simulink model "flightController"  (R2021a)
settings: Solver=ode3  StartTime=0  StopTime=TFinal  FixedStep=Ts  RelTol=1e-3  EnableMultiTasking=on
undefined symbols (not defined in the file): Controller, DiscIntNeverNeededParam, g, K, KLQI, KLQR, linsys, NBar, Ts, Vehicle
settings Model: ExtModeTrigDuration=80  Creator=The MathWorks, Inc.  LastModifiedBy=House
settings SolverCC: AlgebraicLoopSolver=TrustRegion  MinimalZcImpactIntegration=on
settings DataIOCC: LimitDataPoints=on  ReturnWorkspaceOutputs=off
settings OptimizationCC: BlockReduction=off  EnhancedBackFolding=on  PassReuseOutputArgsAs=Individual arguments  ZeroExternalMemoryAtStartup=off  ZeroInternalMemoryAtStartup=off  MaxStackSize=64  OptimizeBlockOrder=speed  DifferentSizesBufferReuse=on  OptimizationCustomize=off  EfficientTunableParamExpr=on
settings DebuggingCC: AlgebraicLoopMsg=none  ParameterPrecisionLossMsg=none  ParameterTunabilityLossMsg=error  UnconnectedInputMsg=none  UnconnectedOutputMsg=none  UnconnectedLineMsg=none  BusObjectLabelMismatch=error  SFUnexpectedBacktrackingDiag=warning  SFNoUnconditionalDefaultTransitionDiag=warning  SFExecutionAtInitializationDiag=none  SFMachineParentedDataDiag=warning  ArithmeticOperatorsInVariantConditions=warning
settings HardwareCC: ProdBitPerPointer=32  ProdBitPerSizeT=32  ProdBitPerPtrDiffT=32  ProdLargestAtomicInteger=Long  ProdWordSize=32  ProdHWDeviceType=ARM Compatible->ARM 9
settings ModelReferenceCC: ModelReferenceNumInstancesAllowed=Single  PropagateSignalLabelsOutOfModel=off
settings SFSimCC: SimUseLocalCustomCode=off  MATLABDynamicMemAlloc=off  CustomCodeUndefinedFunction=UseInterfaceOnly
settings RTWCC: SystemTargetFile=ert.tlc  HardwareBoard=PARROT Mambo  TemplateMakefile=ert_default_tmf  GenerateReport=on  RTWUseLocalCustomCode=off  Toolchain=Sourcery G++ Lite GNU Toolchain for Drones  LaunchReport=on
settings CodeAppCC: ForceParamTrailComments=on  IgnoreCustomStorageClasses=off  MaxIdLength=63  OperatorAnnotations=on  SimulinkDataObjDesc=on  SFDataObjDesc=on  InsertBlockDesc=on
settings ERTTargetCC: MatFileLogging=on
settings ConfigComp: CovMetricSettings=dw  CovSaveCumulativeToWorkspaceVar=on  CovSaveSingleToWorkspaceVar=on  CovExternalEMLEnable=off  CovSFcnEnable=off

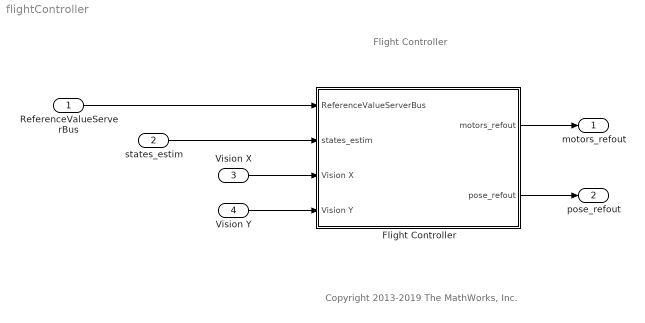
== system flightController ==
  note: Flight Controller
  note: Copyright 2013-2019 The MathWorks, Inc.
  ReferenceValueServerBus : Inport  OutDataTypeStr=Bus: CommandBus  BusOutputAsStruct=on
  states_estim : Inport  Port=2  OutDataTypeStr=Bus: statesEstim_t  BusOutputAsStruct=on
  Vision X : Inport  Port=3
  Vision Y : Inport  Port=4
  Flight Controller : Subsystem
  motors_refout : Outport  VectorParamsAs1DForOutWhenUnconnected=off
  pose_refout : Outport  Port=2  VectorParamsAs1DForOutWhenUnconnected=off
  wires:
  ReferenceValueServerBus/1 -> Flight Controller/1(ReferenceValueServerBus)
  states_estim/1 -> Flight Controller/2(states_estim)
  Flight Controller/2(pose_refout) -> pose_refout/1
  Flight Controller/1(motors_refout) -> motors_refout/1
  Vision X/1 -> Flight Controller/3(Vision X)
  Vision Y/1 -> Flight Controller/4(Vision Y)

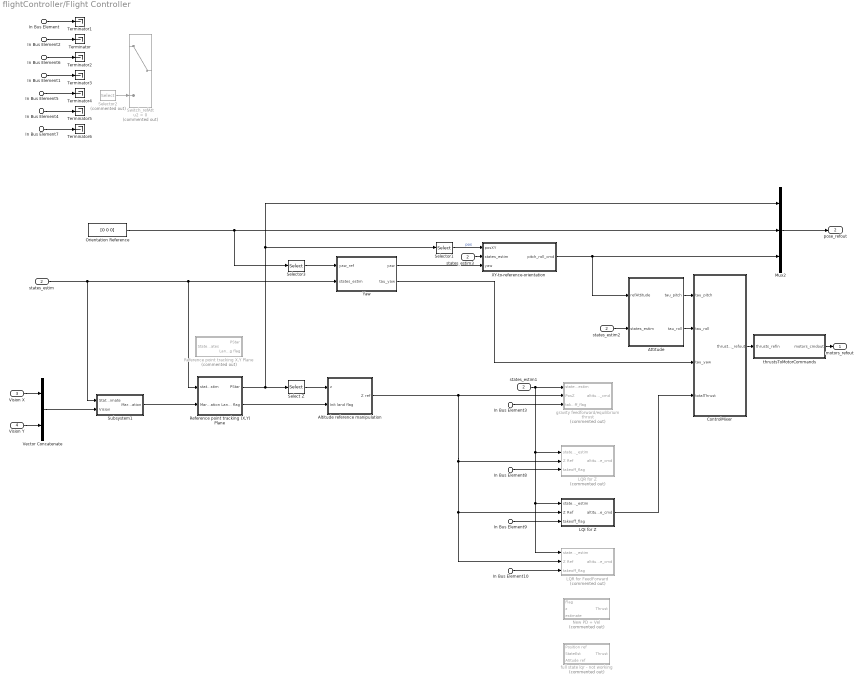
== system flightController/Flight Controller ==
  In Bus Element1 : Inport  PortName=ReferenceValueServerBus  Element=controlModePosVSOrient
  In Bus Element : Inport  PortName=ReferenceValueServerBus  Element=pos_ref
  In Bus Element4 : Inport  PortName=ReferenceValueServerBus  Element=pos_ref
  In Bus Element5 : Inport  PortName=ReferenceValueServerBus  Element=pos_ref
  In Bus Element2 : Inport  PortName=ReferenceValueServerBus  Element=orient_ref
  In Bus Element6 : Inport  PortName=ReferenceValueServerBus  Element=orient_ref
  In Bus Element7 : Inport  PortName=ReferenceValueServerBus  Element=orient_ref
  In Bus Element{3,8..10} (4 alike) : Inport  PortName=ReferenceValueServerBus  Element=takeoff_flag
  states_estim : Inport  Port=2
  Vision X : Inport  Port=3
  Vision Y : Inport  Port=4
  Altitude reference manipulation : Subsystem
  Attitude : Subsystem
  ControlMixer : Subsystem
  LQI for Z : Subsystem
  LQR for FeedForward : Subsystem  Commented=on
  LQR for Z : Subsystem  Commented=on
  Mux2 : Mux  Inputs=3
  New PD + Vel : Subsystem  Commented=on
  Orientation Reference : Constant  Value=[0 0 0]  OutDataTypeStr=single
  Reference point tracking (X,Y) Plane : Subsystem
  Reference point tracking X,Y Plane : Subsystem  Commented=on
  Select Z : Selector  InputPortWidth=3  IndexOptions=Index vector (dialog)  Indices=3  OutputSizes=1
  Selector1 : Selector  InputPortWidth=3  IndexOptions=Index vector (dialog)  Indices=[1 2]  OutputSizes=1
  Selector2 : Selector  Commented=on  InputPortWidth=3  IndexOptions=Index vector (dialog)  Indices=[2 3]  OutputSizes=1
  Selector3 : Selector  InputPortWidth=3  IndexOptions=Index vector (dialog)  Indices=1  OutputSizes=1
  Subsystem1 : Subsystem
  Switch_refAtt : Switch  Commented=on  Criteria=u2 > Threshold
  Terminator{,1..6} (7 alike) : Terminator
  Vector Concatenate : Concatenate
  XY-to-reference-orientation : Subsystem
  Yaw : Subsystem
  full state lqr - not working : Subsystem  Commented=on
  gravity feedforward/equilibrium thrust : Subsystem  Commented=on
  states_estim1 : InportShadow  Port=2
  states_estim2 : InportShadow  Port=2
  states_estim3 : InportShadow  Port=2
  thrustsToMotorCommands : Subsystem
  motors_refout : Outport  VectorParamsAs1DForOutWhenUnconnected=off
  pose_refout : Outport  Port=2  VectorParamsAs1DForOutWhenUnconnected=off
  wires:
  thrustsToMotorCommands/1(motors_cmdout) -> motors_refout/1
  Selector3/1 -> Yaw/1(yaw_ref)
  Selector1/1 -> XY-to-reference-orientation/1(posXY)  "pos"
  ControlMixer/1(thrusts_refout) -> thrustsToMotorCommands/1(thrusts_refin)
  In Bus Element3/1 -> gravity feedforward/equilibrium thrust/3(takeoff_flag)
  states_estim/1 -> Subsystem1/1(State Estimate), Reference point tracking (X,Y) Plane/1(states_estim), Yaw/2(states_estim)
  Yaw/1(yaw) -> XY-to-reference-orientation/3(yaw)
  Mux2/1 -> pose_refout/1
  Attitude/1(tau_pitch) -> ControlMixer/1(tau_pitch)
  Attitude/2(tau_roll) -> ControlMixer/2(tau_roll)
  Yaw/2(tau_yaw) -> ControlMixer/3(tau_yaw)
  states_estim1/1 -> LQR for FeedForward/1(states_estim), LQI for Z/1(states_estim), LQR for Z/1(states_estim), gravity feedforward/equilibrium thrust/1(states_estim)
  states_estim2/1 -> Attitude/2(states_estim)
  states_estim3/1 -> XY-to-reference-orientation/2(states_estim)
  Selector2/1 -> Switch_refAtt/3
  In Bus Element2/1 -> Terminator/1
  In Bus Element/1 -> Terminator1/1
  In Bus Element6/1 -> Terminator2/1
  In Bus Element1/1 -> Terminator3/1
  In Bus Element5/1 -> Terminator4/1
  XY-to-reference-orientation/1(pitch_roll_cmd) -> Attitude/1(refAttitude), Mux2/3
  In Bus Element4/1 -> Terminator5/1
  Orientation Reference/1 -> Selector3/1, Mux2/2
  In Bus Element7/1 -> Terminator6/1
  Altitude reference manipulation/1(Z ref) -> LQR for FeedForward/2(Z Ref), LQI for Z/2(Z Ref), LQR for Z/2(Z Ref), gravity feedforward/equilibrium thrust/2(PosZ)
  In Bus Element8/1 -> LQR for Z/3(takeoff_flag)
  In Bus Element9/1 -> LQI for Z/3(takeoff_flag)
  In Bus Element10/1 -> LQR for FeedForward/3(takeoff_flag)
  Select Z/1 -> Altitude reference manipulation/1(z)
  Reference point tracking (X,Y) Plane/1(PStar) -> Selector1/1, Mux2/1, Select Z/1
  Reference point tracking (X,Y) Plane/2(Landing flag) -> Altitude reference manipulation/2(Init land flag)
  Vision X/1 -> Vector Concatenate/1
  Vision Y/1 -> Vector Concatenate/2
  Vector Concatenate/1 -> Subsystem1/2(Vision)
  Subsystem1/1(Marker Location) -> Reference point tracking (X,Y) Plane/2(Marker Location)
  LQI for Z/1(altitude_cmd) -> ControlMixer/4(totalThrust)

== system flightController/Flight Controller/Altitude reference manipulation ==
  z : Inport
  Init land flag : Inport  Port=2
  Constant3 : Constant  Value=Ts  OutDataTypeStr=single
  Delay : Delay  DelayLength=600
  Landing spline : Scope  NumInputPorts=2
  Landing spline Dependent on time - works : MATLAB Function  TreatAsAtomicUnit=on
  Landing spline Dependent on time - works My version : MATLAB Function  Commented=on  TreatAsAtomicUnit=on
  Memory : Memory
  Switch : Switch  Criteria=u2 > Threshold
  Z ref : Outport
  wires:
  Constant3/1 -> Landing spline Dependent on time - works/2(time)
  Delay/1 -> Landing spline Dependent on time - works/3(flag)
  Landing spline Dependent on time - works/1(ZdOut) -> Landing spline/2, Z ref/1
  Init land flag/1 -> Switch/2, Delay/1
  z/1 -> Switch/3
  Switch/1 -> Memory/1, Landing spline/1, Landing spline Dependent on time - works/1(z)
  Memory/1 -> Switch/1

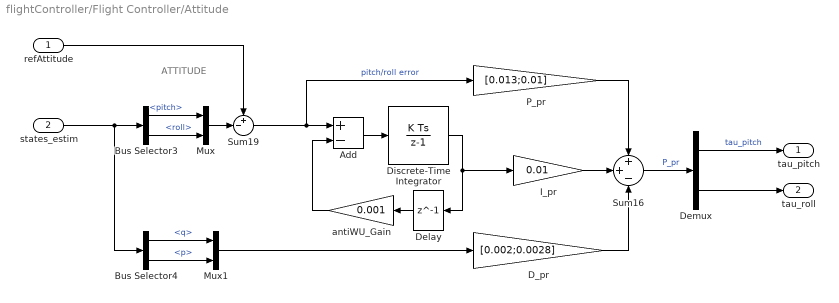
== system flightController/Flight Controller/Attitude ==
  note: ATTITUDE
  refAttitude : Inport
  states_estim : Inport  Port=2
  Add : Sum  Inputs=+-
  Bus Selector3 : BusSelector  OutputSignals=pitch,roll
  Bus Selector4 : BusSelector  OutputSignals=q,p
  D_pr : Gain  Gain=[0.002;0.0028]
  Delay : Delay  DelayLength=1  InitialCondition=0
  Demux : Demux  Outputs=2
  Discrete-Time Integrator : DiscreteIntegrator  SampleTime=Ts  LimitOutput=on  UpperSaturationLimit=2  LowerSaturationLimit=-2  ICPrevOutput=DiscIntNeverNeededParam  ICPrevScaledInput=DiscIntNeverNeededParam
  I_pr : Gain  Gain=0.01
  Mux : Mux  Inputs=2
  Mux1 : Mux  Inputs=2
  P_pr : Gain  Gain=[0.013;0.01]
  Sum16 : Sum  Inputs=++-  AccumDataTypeStr=single  OutDataTypeStr=single  SaturateOnIntegerOverflow=on
  Sum19 : Sum  Inputs=+-|
  antiWU_Gain : Gain  Gain=0.001
  tau_pitch : Outport  VectorParamsAs1DForOutWhenUnconnected=off
  tau_roll : Outport  Port=2  VectorParamsAs1DForOutWhenUnconnected=off
  wires:
  Sum16/1 -> Demux/1  "P_pr"
  antiWU_Gain/1 -> Add/2
  Add/1 -> Discrete-Time Integrator/1
  Bus Selector3/1 -> Mux/1  "<pitch>"
  Bus Selector4/1 -> Mux1/1  "<q>"
  P_pr/1 -> Sum16/1
  I_pr/1 -> Sum16/2
  Sum19/1 -> Add/1, P_pr/1  "pitch/roll error"
  Discrete-Time Integrator/1 -> Delay/1, I_pr/1
  Delay/1 -> antiWU_Gain/1
  Demux/1 -> tau_pitch/1  "tau_pitch"
  Demux/2 -> tau_roll/1
  D_pr/1 -> Sum16/3
  states_estim/1 -> Bus Selector3/1, Bus Selector4/1
  refAttitude/1 -> Sum19/1
  Mux/1 -> Sum19/2
  Bus Selector3/2 -> Mux/2  "<roll>"
  Mux1/1 -> D_pr/1
  Bus Selector4/2 -> Mux1/2  "<p>"

== system flightController/Flight Controller/ControlMixer ==
  tau_pitch : Inport
  tau_roll : Inport  Port=2
  tau_yaw : Inport  Port=3
  totalThrust : Inport  Port=4
  Mux2 : Mux
  Product : Product  Multiplication=Matrix(*)  RndMeth=Zero
  TorqueTotalThrustToThrustPerMotor : Constant  Value=Controller.Q2Ts  OutDataTypeStr=single
  thrusts_refout : Outport  VectorParamsAs1DForOutWhenUnconnected=off
  wires:
  Product/1 -> thrusts_refout/1
  tau_roll/1 -> Mux2/4
  tau_pitch/1 -> Mux2/3
  tau_yaw/1 -> Mux2/2
  totalThrust/1 -> Mux2/1
  TorqueTotalThrustToThrustPerMotor/1 -> Product/1
  Mux2/1 -> Product/2

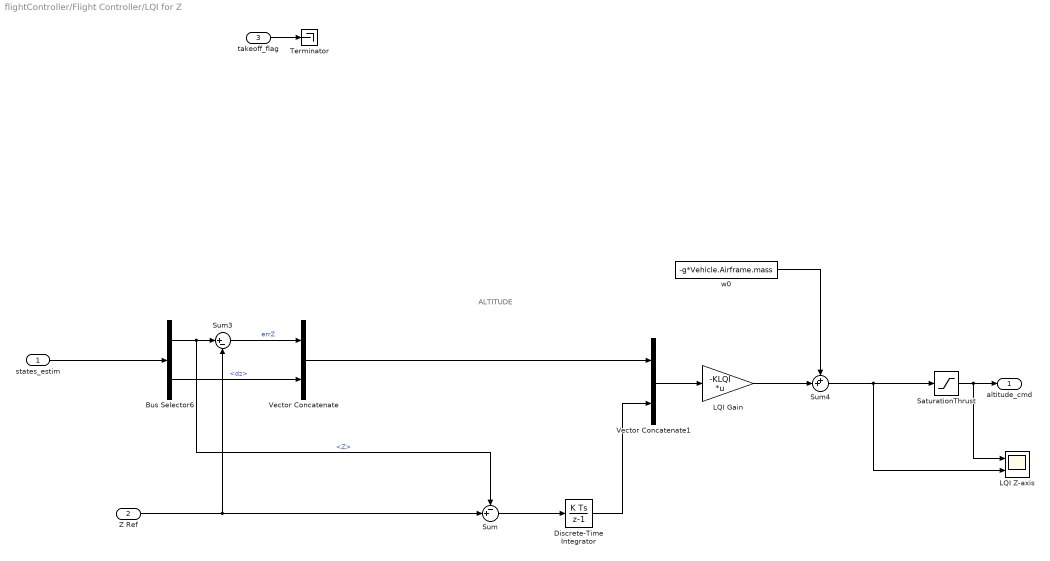
== system flightController/Flight Controller/LQI for Z ==
  note: ALTITUDE
  states_estim : Inport
  Z Ref : Inport  Port=2
  takeoff_flag : Inport  Port=3
  Bus Selector6 : BusSelector  OutputSignals=Z,dz
  Discrete-Time Integrator : DiscreteIntegrator  SampleTime=-1  ICPrevOutput=DiscIntNeverNeededParam  ICPrevScaledInput=DiscIntNeverNeededParam
  LQI Gain : Gain  Gain=-KLQI  Multiplication=Matrix(K*u) (u vector)
  LQI Z-axis : Scope  NumInputPorts=2
  SaturationThrust : Saturate  UpperLimit=4*Controller.totalThrustMaxRelative*Controller.motorsThrustPerMotorMax  LowerLimit=-4*Controller.totalThrustMaxRelative*Controller.motorsThrustPerMotorMax  OutDataTypeStr=single
  Sum : Sum  Inputs=-+|
  Sum3 : Sum  Inputs=|+-  AccumDataTypeStr=single  OutDataTypeStr=single  SaturateOnIntegerOverflow=on
  Sum4 : Sum  Inputs=++|  AccumDataTypeStr=single  OutDataTypeStr=single  SaturateOnIntegerOverflow=on
  Terminator : Terminator
  Vector Concatenate : Concatenate
  Vector Concatenate1 : Concatenate
  w0 : Constant  Value=-g*Vehicle.Airframe.mass  OutDataTypeStr=single  SampleTime=Ts
  altitude_cmd : Outport  VectorParamsAs1DForOutWhenUnconnected=off
  wires:
  states_estim/1 -> Bus Selector6/1
  Sum4/1 -> LQI Z-axis/2, SaturationThrust/1
  w0/1 -> Sum4/1
  SaturationThrust/1 -> LQI Z-axis/1, altitude_cmd/1
  Bus Selector6/2 -> Vector Concatenate/2  "<dz>"
  takeoff_flag/1 -> Terminator/1
  Sum3/1 -> Vector Concatenate/1  "errZ"
  LQI Gain/1 -> Sum4/2
  Vector Concatenate1/1 -> LQI Gain/1
  Vector Concatenate/1 -> Vector Concatenate1/1
  Discrete-Time Integrator/1 -> Vector Concatenate1/2
  Z Ref/1 -> Sum3/2, Sum/2
  Sum/1 -> Discrete-Time Integrator/1
  Bus Selector6/1 -> Sum/1, Sum3/1  "<Z>"

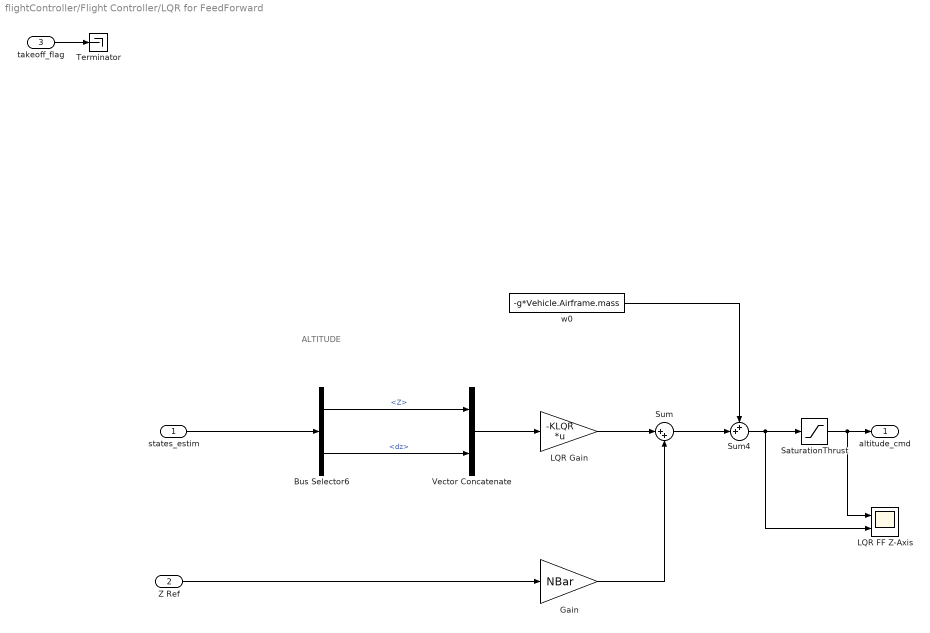
== system flightController/Flight Controller/LQR for FeedForward ==
  note: ALTITUDE
  states_estim : Inport
  Z Ref : Inport  Port=2
  takeoff_flag : Inport  Port=3
  Bus Selector6 : BusSelector  OutputSignals=Z,dz
  Gain : Gain  Gain=NBar
  LQR FF Z-Axis : Scope  NumInputPorts=2
  LQR Gain : Gain  Gain=-KLQR  Multiplication=Matrix(K*u) (u vector)
  SaturationThrust : Saturate  UpperLimit=4*Controller.totalThrustMaxRelative*Controller.motorsThrustPerMotorMax  LowerLimit=-4*Controller.totalThrustMaxRelative*Controller.motorsThrustPerMotorMax  OutDataTypeStr=single
  Sum : Sum  Inputs=|++
  Sum4 : Sum  Inputs=++|  AccumDataTypeStr=single  OutDataTypeStr=single  SaturateOnIntegerOverflow=on
  Terminator : Terminator
  Vector Concatenate : Concatenate
  w0 : Constant  Value=-g*Vehicle.Airframe.mass  OutDataTypeStr=single  SampleTime=Ts
  altitude_cmd : Outport  VectorParamsAs1DForOutWhenUnconnected=off
  wires:
  states_estim/1 -> Bus Selector6/1
  Sum4/1 -> LQR FF Z-Axis/2, SaturationThrust/1
  SaturationThrust/1 -> LQR FF Z-Axis/1, altitude_cmd/1
  Bus Selector6/2 -> Vector Concatenate/2  "<dz>"
  takeoff_flag/1 -> Terminator/1
  Vector Concatenate/1 -> LQR Gain/1
  Z Ref/1 -> Gain/1
  Bus Selector6/1 -> Vector Concatenate/1  "<Z>"
  w0/1 -> Sum4/1
  LQR Gain/1 -> Sum/1
  Sum/1 -> Sum4/2
  Gain/1 -> Sum/2

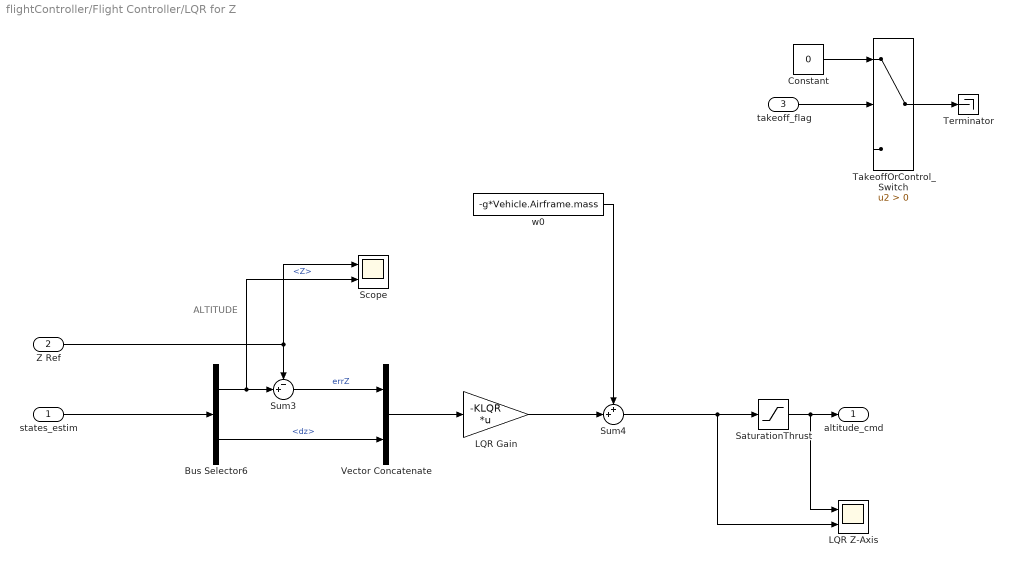
== system flightController/Flight Controller/LQR for Z ==
  note: ALTITUDE
  states_estim : Inport
  Z Ref : Inport  Port=2
  takeoff_flag : Inport  Port=3
  Bus Selector6 : BusSelector  OutputSignals=Z,dz
  Constant : Constant  Value=0  OutDataTypeStr=single
  LQR Gain : Gain  Gain=-KLQR  Multiplication=Matrix(K*u) (u vector)
  LQR Z-Axis : Scope  NumInputPorts=2
  SaturationThrust : Saturate  UpperLimit=4*Controller.totalThrustMaxRelative*Controller.motorsThrustPerMotorMax  LowerLimit=-4*Controller.totalThrustMaxRelative*Controller.motorsThrustPerMotorMax  OutDataTypeStr=single
  Scope : Scope  NumInputPorts=2
  Sum3 : Sum  Inputs=-+|  AccumDataTypeStr=single  OutDataTypeStr=single  SaturateOnIntegerOverflow=on
  Sum4 : Sum  Inputs=++|  AccumDataTypeStr=single  OutDataTypeStr=single  SaturateOnIntegerOverflow=on
  TakeoffOrControl_Switch : Switch  Criteria=u2 > Threshold
  Terminator : Terminator
  Vector Concatenate : Concatenate
  w0 : Constant  Value=-g*Vehicle.Airframe.mass  OutDataTypeStr=single  SampleTime=Ts
  altitude_cmd : Outport  VectorParamsAs1DForOutWhenUnconnected=off
  wires:
  states_estim/1 -> Bus Selector6/1
  Sum4/1 -> LQR Z-Axis/2, SaturationThrust/1
  w0/1 -> Sum4/1
  SaturationThrust/1 -> altitude_cmd/1, LQR Z-Axis/1
  Bus Selector6/2 -> Vector Concatenate/2  "<dz>"
  Bus Selector6/1 -> Scope/2, Sum3/2  "<Z>"
  Z Ref/1 -> Sum3/1, Scope/1
  Sum3/1 -> Vector Concatenate/1  "errZ"
  Vector Concatenate/1 -> LQR Gain/1
  LQR Gain/1 -> Sum4/2
  Constant/1 -> TakeoffOrControl_Switch/1
  takeoff_flag/1 -> TakeoffOrControl_Switch/2
  TakeoffOrControl_Switch/1 -> Terminator/1

== system flightController/Flight Controller/New PD + Vel ==
  Flag : Inport
  z : Inport  Port=2
  estimate : Inport  Port=3
  Altitude reference manipulation With Velocity calculation : Subsystem
  gravity feedforward/equilibrium thrust : Subsystem
  Thrust : Outport
  wires:
  Flag/1 -> Altitude reference manipulation With Velocity calculation/1(Init land flag)
  z/1 -> Altitude reference manipulation With Velocity calculation/2(z)
  estimate/1 -> gravity feedforward/equilibrium thrust/1(states_estim), Altitude reference manipulation With Velocity calculation/3(State estimate)
  Altitude reference manipulation With Velocity calculation/1(Z ref) -> gravity feedforward/equilibrium thrust/2(PosZ)
  gravity feedforward/equilibrium thrust/1(altitude_cmd) -> Thrust/1

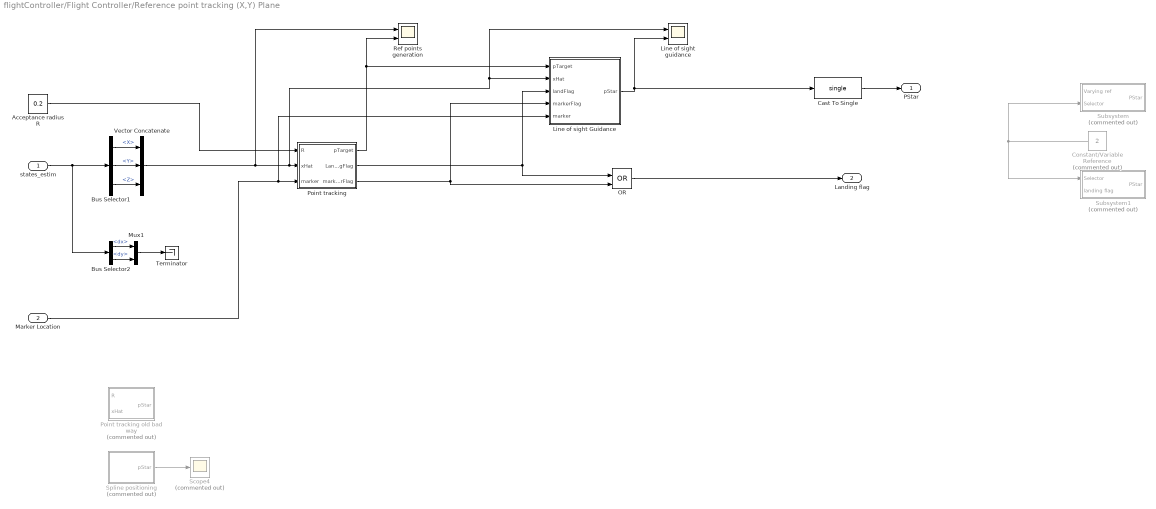
== system flightController/Flight Controller/Reference point tracking (X,Y) Plane ==
  states_estim : Inport
  Marker Location : Inport  Port=2
  Acceptance radius R : Constant  Value=0.2  OutDataTypeStr=single
  Bus Selector1 : BusSelector  OutputSignals=X,Y,Z
  Bus Selector2 : BusSelector  OutputSignals=dx,dy
  Cast To Single : DataTypeConversion  OutDataTypeStr=single
  Constant/Variable Reference : Constant  Commented=on  Value=2  OutDataTypeStr=single
  Line of sight Guidance : MATLAB Function  TreatAsAtomicUnit=on
  Line of sight guidance : Scope  NumInputPorts=2
  Mux1 : Mux  Inputs=2
  OR : Logic  Operator=OR  IconShape=distinctive  AllPortsSameDT=off  OutDataTypeStr=boolean
  Point tracking : MATLAB Function  TreatAsAtomicUnit=on
  Point tracking old bad way : MATLAB Function  Commented=on  TreatAsAtomicUnit=on
  Ref points generation : Scope  NumInputPorts=2
  Scope4 : Scope  Commented=on
  Spline positioning : MATLAB Function  Commented=on  TreatAsAtomicUnit=on
  Subsystem : Subsystem  Commented=on
  Subsystem1 : Subsystem  Commented=on
  Terminator : Terminator
  Vector Concatenate : Concatenate  NumInputs=3
  PStar : Outport
  Landing flag : Outport  Port=2
  wires:
  Bus Selector2/1 -> Mux1/1  "<dx>"
  states_estim/1 -> Bus Selector2/1, Bus Selector1/1
  Bus Selector1/2 -> Vector Concatenate/2  "<Y>"
  Bus Selector1/3 -> Vector Concatenate/3  "<Z>"
  Bus Selector1/1 -> Vector Concatenate/1  "<X>"
  Bus Selector2/2 -> Mux1/2  "<dy>"
  Mux1/1 -> Terminator/1
  Spline positioning/1(pStar) -> Scope4/1
  Line of sight Guidance/1(pStar) -> Cast To Single/1, Line of sight guidance/2
  Constant/Variable Reference/1 -> Subsystem1/1(Selector), Subsystem/2(Selector)
  Cast To Single/1 -> PStar/1
  Point tracking/1(pTarget) -> Ref points generation/2, Line of sight Guidance/1(pTarget)
  Vector Concatenate/1 -> Ref points generation/1, Line of sight guidance/1, Line of sight Guidance/2(xHat), Point tracking/2(xHat)
  Acceptance radius R/1 -> Point tracking/1(R)
  Point tracking/2(LandingFlag) -> OR/1, Line of sight Guidance/3(landFlag)
  Marker Location/1 -> Line of sight Guidance/5(marker), Point tracking/3(marker)
  Point tracking/3(markerFlag) -> OR/2, Line of sight Guidance/4(markerFlag)
  OR/1 -> Landing flag/1

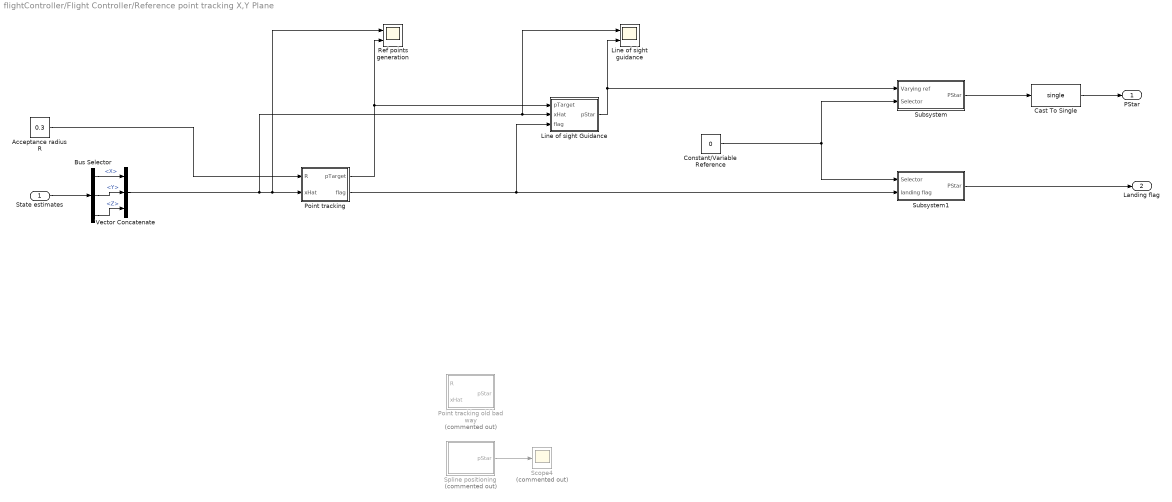
== system flightController/Flight Controller/Reference point tracking X,Y Plane ==
  State estimates : Inport
  Acceptance radius R : Constant  Value=0.3
  Bus Selector : BusSelector  OutputSignals=X,Y,Z
  Cast To Single : DataTypeConversion  OutDataTypeStr=single
  Constant/Variable Reference : Constant  Value=0
  Line of sight Guidance : MATLAB Function  TreatAsAtomicUnit=on
  Line of sight guidance : Scope  NumInputPorts=2
  Point tracking : MATLAB Function  TreatAsAtomicUnit=on
  Point tracking old bad way : MATLAB Function  Commented=on  TreatAsAtomicUnit=on
  Ref points generation : Scope  NumInputPorts=2
  Scope4 : Scope  Commented=on
  Spline positioning : MATLAB Function  Commented=on  TreatAsAtomicUnit=on
  Subsystem : Subsystem
  Subsystem1 : Subsystem
  Vector Concatenate : Concatenate  NumInputs=3
  PStar : Outport
  Landing flag : Outport  Port=2
  wires:
  Bus Selector/3 -> Vector Concatenate/3  "<Z>"
  Bus Selector/1 -> Vector Concatenate/1  "<X>"
  Point tracking/1(pTarget) -> Line of sight Guidance/1(pTarget), Ref points generation/2
  Acceptance radius R/1 -> Point tracking/1(R)
  Bus Selector/2 -> Vector Concatenate/2  "<Y>"
  Vector Concatenate/1 -> Line of sight guidance/1, Line of sight Guidance/2(xHat), Ref points generation/1, Point tracking/2(xHat)
  Line of sight Guidance/1(pStar) -> Subsystem/1(Varying ref), Line of sight guidance/2
  Point tracking/2(flag) -> Subsystem1/2(landing flag), Line of sight Guidance/3(flag)
  State estimates/1 -> Bus Selector/1
  Spline positioning/1(pStar) -> Scope4/1
  Constant/Variable Reference/1 -> Subsystem1/1(Selector), Subsystem/2(Selector)
  Subsystem/1(PStar) -> Cast To Single/1
  Subsystem1/1(PStar) -> Landing flag/1
  Cast To Single/1 -> PStar/1

== system flightController/Flight Controller/Subsystem1 ==
  State Estimate : Inport
  Vision : Inport  Port=2
  Bus Selector6 : BusSelector  OutputSignals=Z
  Constant : Constant  Value=0.004  OutDataTypeStr=single
  Display : Display
  Display1 : Display
  Display2 : Display
  Divide : Product  Inputs=**
  Divide1 : Product  Inputs=**
  Gain : Gain  OutDataTypeStr=Inherit: Same as input
  Marker Location : Outport
  wires:
  State Estimate/1 -> Bus Selector6/1
  Bus Selector6/1 -> Divide/2, Display2/1  "<Z>"
  Constant/1 -> Divide/1
  Divide/1 -> Divide1/2
  Vision/1 -> Display/1, Divide1/1
  Divide1/1 -> Gain/1
  Gain/1 -> Display1/1, Marker Location/1

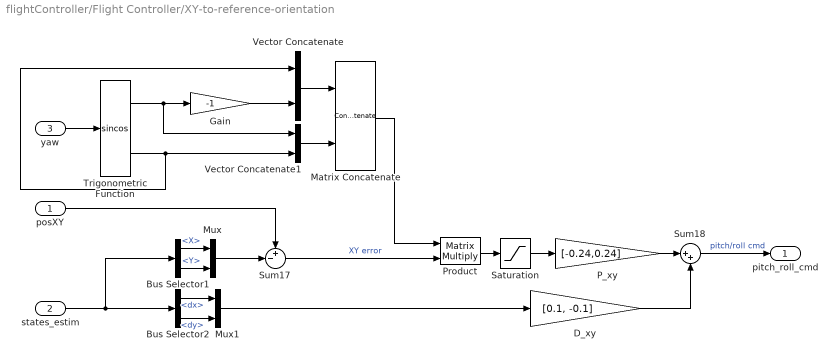
== system flightController/Flight Controller/XY-to-reference-orientation ==
  posXY : Inport
  states_estim : Inport  Port=2
  yaw : Inport  Port=3
  Bus Selector1 : BusSelector  OutputSignals=X,Y
  Bus Selector2 : BusSelector  OutputSignals=dx,dy
  D_xy : Gain  Gain=[0.1, -0.1]  ParamDataTypeStr=single  OutDataTypeStr=single  SaturateOnIntegerOverflow=on
  Gain : Gain  Gain=-1
  Matrix Concatenate : Concatenate  Mode=Multidimensional array  ConcatenateDimension=2
  Mux : Mux  Inputs=2
  Mux1 : Mux  Inputs=2
  P_xy : Gain  Gain=[-0.24,0.24]  ParamDataTypeStr=single  OutDataTypeStr=single  SaturateOnIntegerOverflow=on
  Product : Product  Multiplication=Matrix(*)  OutDataTypeStr=single  RndMeth=Zero
  Saturation : Saturate  UpperLimit=3  LowerLimit=-3  OutDataTypeStr=single
  Sum17 : Sum  Inputs=+-|  AccumDataTypeStr=single
  Sum18 : Sum  Inputs=|++  AccumDataTypeStr=single  OutDataTypeStr=single  SaturateOnIntegerOverflow=on
  Trigonometric Function : Trigonometry  Operator=sincos
  Vector Concatenate : Concatenate
  Vector Concatenate1 : Concatenate
  pitch_roll_cmd : Outport  VectorParamsAs1DForOutWhenUnconnected=off
  wires:
  yaw/1 -> Trigonometric Function/1
  Saturation/1 -> P_xy/1
  P_xy/1 -> Sum18/1
  Sum17/1 -> Product/2  "XY error"
  posXY/1 -> Sum17/1
  Bus Selector2/1 -> Mux1/1  "<dx>"
  states_estim/1 -> Bus Selector1/1, Bus Selector2/1
  Sum18/1 -> pitch_roll_cmd/1  "pitch/roll cmd"
  D_xy/1 -> Sum18/2
  Bus Selector1/1 -> Mux/1  "<X>"
  Product/1 -> Saturation/1
  Trigonometric Function/1 -> Gain/1, Vector Concatenate1/1
  Trigonometric Function/2 -> Vector Concatenate1/2, Vector Concatenate/1
  Gain/1 -> Vector Concatenate/2
  Vector Concatenate/1 -> Matrix Concatenate/1
  Vector Concatenate1/1 -> Matrix Concatenate/2
  Matrix Concatenate/1 -> Product/1
  Bus Selector1/2 -> Mux/2  "<Y>"
  Mux/1 -> Sum17/2
  Mux1/1 -> D_xy/1
  Bus Selector2/2 -> Mux1/2  "<dy>"

== system flightController/Flight Controller/Yaw ==
  yaw_ref : Inport
  states_estim : Inport  Port=2
  Bus Selector5 : BusSelector  OutputSignals=yaw,r
  D_yaw : Gain  Gain=0.3*0.004
  P_yaw : Gain  Gain=0.004  ParamDataTypeStr=single  OutDataTypeStr=single
  Sum1 : Sum  Inputs=+-|  AccumDataTypeStr=single  OutDataTypeStr=single  SaturateOnIntegerOverflow=on
  Sum2 : Sum  Inputs=|+-
  yaw : Outport  VectorParamsAs1DForOutWhenUnconnected=off
  tau_yaw : Outport  Port=2  VectorParamsAs1DForOutWhenUnconnected=off
  wires:
  D_yaw/1 -> Sum2/2
  P_yaw/1 -> Sum2/1
  Bus Selector5/2 -> D_yaw/1  "<r>"
  Sum1/1 -> P_yaw/1
  states_estim/1 -> Bus Selector5/1
  Sum2/1 -> tau_yaw/1
  Bus Selector5/1 -> yaw/1, Sum1/2  "<yaw>"
  yaw_ref/1 -> Sum1/1

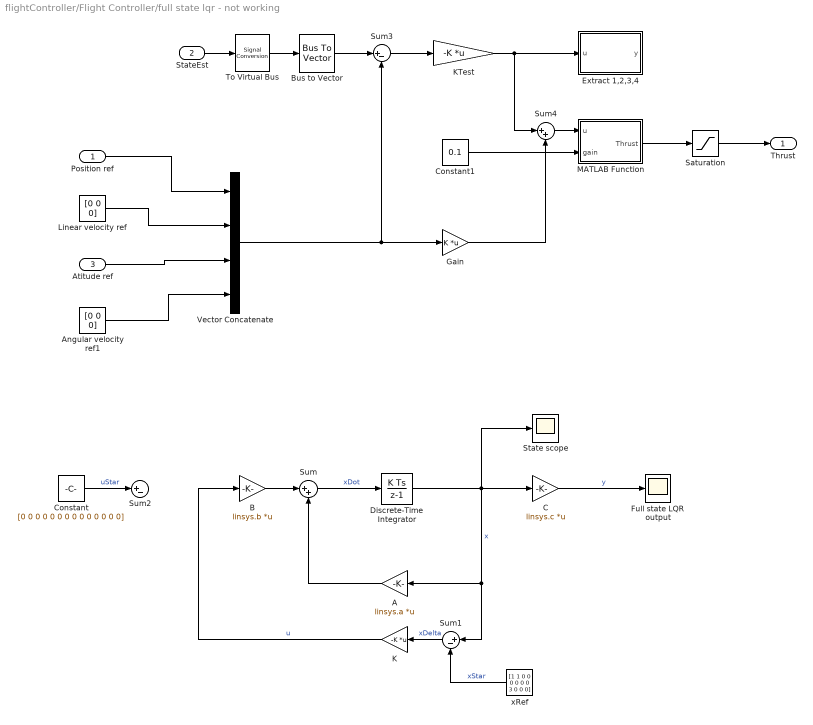
== system flightController/Flight Controller/full state lqr - not working ==
  Position ref : Inport
  StateEst : Inport  Port=2
  Atitude ref : Inport  Port=3
  A : Gain  Gain=linsys.a  Multiplication=Matrix(K*u) (u vector)
  Angular velocity ref1 : Constant  Value=[0 0 0]  OutDataTypeStr=single
  B : Gain  Gain=linsys.b  Multiplication=Matrix(K*u) (u vector)
  Bus to Vector : BusToVector
  C : Gain  Gain=linsys.c  Multiplication=Matrix(K*u) (u vector)
  Constant : Constant  Value=[0 0 0 0 0 0 0 0 0 0 0 0 0 0]
  Constant1 : Constant  Value=0.1
  Discrete-Time Integrator : DiscreteIntegrator  InitialCondition=[0 0 0 0 0 0 0 0 0 0 0 0]  SampleTime=-1  ICPrevOutput=DiscIntNeverNeededParam  ICPrevScaledInput=DiscIntNeverNeededParam
  Extract 1,2,3,4 : MATLAB Function  TreatAsAtomicUnit=on
  Full state LQR output : Scope
  Gain : Gain  Gain=K  Multiplication=Matrix(K*u) (u vector)
  K : Gain  Gain=-K  Multiplication=Matrix(K*u) (u vector)
  KTest : Gain  Gain=-K  Multiplication=Matrix(K*u) (u vector)
  Linear velocity ref : Constant  Value=[0 0 0]  OutDataTypeStr=single
  MATLAB Function : MATLAB Function  TreatAsAtomicUnit=on
  Saturation : Saturate  UpperLimit=1  LowerLimit=-1
  State scope : Scope
  Sum : Sum  Inputs=|++
  Sum1 : Sum  Inputs=|+-
  Sum2 : Sum  Inputs=|+-
  Sum3 : Sum  Inputs=|+-
  Sum4 : Sum  Inputs=|++
  To Virtual Bus : SignalConversion  ConversionOutput=Virtual bus  OverrideOpt=off
  Vector Concatenate : Concatenate  NumInputs=4
  xRef : Constant  Value=[1 1 0 0 0 0 0 0 3 0 0 0]
  Thrust : Outport
  wires:
  StateEst/1 -> To Virtual Bus/1
  To Virtual Bus/1 -> Bus to Vector/1
  B/1 -> Sum/1
  A/1 -> Sum/2
  Sum/1 -> Discrete-Time Integrator/1  "xDot"
  Discrete-Time Integrator/1 -> State scope/1, A/1, Sum1/1, C/1  "x"
  K/1 -> B/1  "u"
  Sum1/1 -> K/1  "xDelta"
  xRef/1 -> Sum1/2  "xStar"
  Constant/1 -> Sum2/1  "uStar"
  C/1 -> Full state LQR output/1  "y"
  Bus to Vector/1 -> Sum3/1
  Sum3/1 -> KTest/1
  Position ref/1 -> Vector Concatenate/1
  Linear velocity ref/1 -> Vector Concatenate/2
  Atitude ref/1 -> Vector Concatenate/3
  Angular velocity ref1/1 -> Vector Concatenate/4
  Vector Concatenate/1 -> Gain/1, Sum3/2
  Constant1/1 -> MATLAB Function/2(gain)
  Sum4/1 -> MATLAB Function/1(u)
  KTest/1 -> Sum4/1, Extract 1,2,3,4/1(u)
  MATLAB Function/1(Thrust) -> Saturation/1
  Saturation/1 -> Thrust/1
  Gain/1 -> Sum4/2

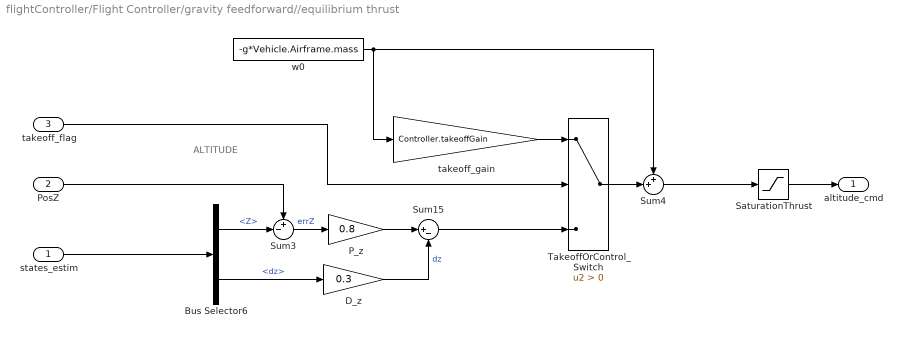
== system flightController/Flight Controller/gravity feedforward//equilibrium thrust ==
  note: ALTITUDE
  states_estim : Inport
  PosZ : Inport  Port=2
  takeoff_flag : Inport  Port=3
  Bus Selector6 : BusSelector  OutputSignals=Z,dz
  D_z : Gain  Gain=0.3  ParamDataTypeStr=single  OutDataTypeStr=single  SaturateOnIntegerOverflow=on
  P_z : Gain  Gain=0.8  ParamDataTypeStr=single  OutDataTypeStr=single  SaturateOnIntegerOverflow=on
  SaturationThrust : Saturate  UpperLimit=4*Controller.totalThrustMaxRelative*Controller.motorsThrustPerMotorMax  LowerLimit=-4*Controller.totalThrustMaxRelative*Controller.motorsThrustPerMotorMax  OutDataTypeStr=single
  Sum15 : Sum  Inputs=|+-  AccumDataTypeStr=single  OutDataTypeStr=single  SaturateOnIntegerOverflow=on
  Sum3 : Sum  Inputs=+-|  AccumDataTypeStr=single  OutDataTypeStr=single  SaturateOnIntegerOverflow=on
  Sum4 : Sum  Inputs=++|  AccumDataTypeStr=single  OutDataTypeStr=single  SaturateOnIntegerOverflow=on
  TakeoffOrControl_Switch : Switch  Criteria=u2 > Threshold
  takeoff_gain : Gain  Gain=Controller.takeoffGain  ParamDataTypeStr=single  OutDataTypeStr=single  SaturateOnIntegerOverflow=on
  w0 : Constant  Value=-g*Vehicle.Airframe.mass  OutDataTypeStr=single  SampleTime=Ts
  altitude_cmd : Outport  VectorParamsAs1DForOutWhenUnconnected=off
  wires:
  Sum3/1 -> P_z/1  "errZ"
  TakeoffOrControl_Switch/1 -> Sum4/2
  Bus Selector6/1 -> Sum3/2  "<Z>"
  Bus Selector6/2 -> D_z/1  "<dz>"
  w0/1 -> Sum4/1, takeoff_gain/1
  D_z/1 -> Sum15/2  "dz"
  takeoff_gain/1 -> TakeoffOrControl_Switch/1
  takeoff_flag/1 -> TakeoffOrControl_Switch/2
  PosZ/1 -> Sum3/1
  P_z/1 -> Sum15/1
  Sum15/1 -> TakeoffOrControl_Switch/3
  Sum4/1 -> SaturationThrust/1
  SaturationThrust/1 -> altitude_cmd/1
  states_estim/1 -> Bus Selector6/1

== system flightController/Flight Controller/thrustsToMotorCommands ==
  thrusts_refin : Inport
  MotorDirections : Gain  Gain=[1 -1 1 -1]
  Saturation5 : Saturate  UpperLimit=Vehicle.Motor.maxLimit  LowerLimit=Vehicle.Motor.minLimit
  ThrustToMotorCommand : Gain  Gain=-Vehicle.Motor.thrustToMotorCommand
  motors_cmdout : Outport  VectorParamsAs1DForOutWhenUnconnected=off
  wires:
  Saturation5/1 -> MotorDirections/1
  MotorDirections/1 -> motors_cmdout/1
  ThrustToMotorCommand/1 -> Saturation5/1
  thrusts_refin/1 -> ThrustToMotorCommand/1

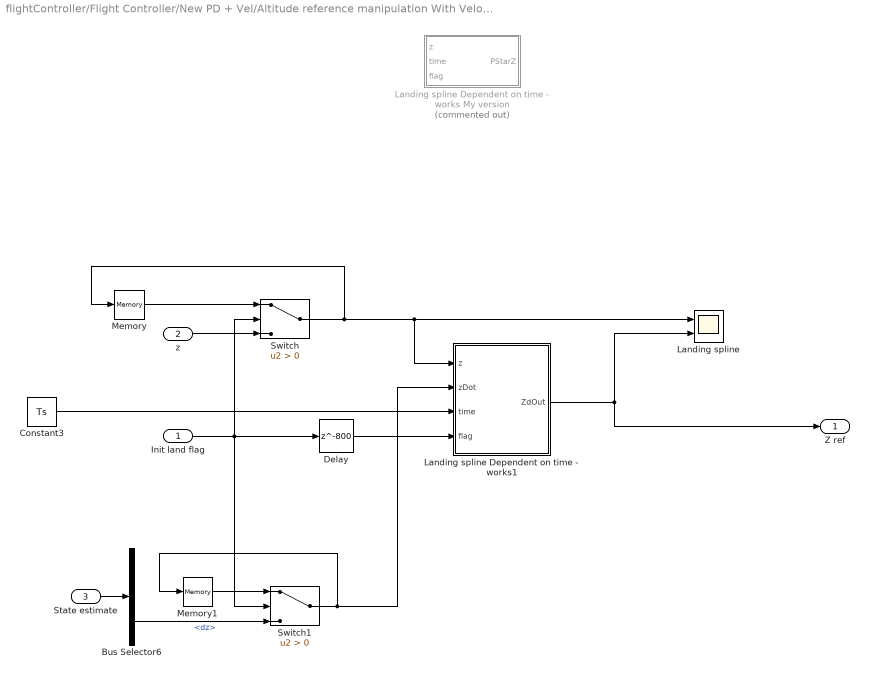
== system flightController/Flight Controller/New PD + Vel/Altitude reference manipulation With Velocity calculation ==
  Init land flag : Inport
  z : Inport  Port=2
  State estimate : Inport  Port=3
  Bus Selector6 : BusSelector  OutputSignals=Z,dz
  Constant3 : Constant  Value=Ts
  Delay : Delay  DelayLength=800
  Landing spline : Scope  NumInputPorts=2
  Landing spline Dependent on time - works My version : MATLAB Function  Commented=on  TreatAsAtomicUnit=on
  Landing spline Dependent on time - works1 : MATLAB Function  TreatAsAtomicUnit=on
  Memory : Memory
  Memory1 : Memory
  Switch : Switch  Criteria=u2 > Threshold
  Switch1 : Switch  Criteria=u2 > Threshold
  Z ref : Outport
  wires:
  Constant3/1 -> Landing spline Dependent on time - works1/3(time)
  Delay/1 -> Landing spline Dependent on time - works1/4(flag)
  Init land flag/1 -> Switch1/2, Switch/2, Delay/1
  z/1 -> Switch/3
  Switch/1 -> Memory/1, Landing spline/1, Landing spline Dependent on time - works1/1(z)
  Memory/1 -> Switch/1
  State estimate/1 -> Bus Selector6/1
  Bus Selector6/2 -> Switch1/3  "<dz>"
  Switch1/1 -> Memory1/1, Landing spline Dependent on time - works1/2(zDot)
  Memory1/1 -> Switch1/1
  Landing spline Dependent on time - works1/1(ZdOut) -> Z ref/1, Landing spline/2

== system flightController/Flight Controller/New PD + Vel/gravity feedforward//equilibrium thrust ==
  note: ALTITUDE
  states_estim : Inport
  PosZ : Inport  Port=2
  Bus Selector6 : BusSelector  OutputSignals=Z,dz
  D_z : Gain  Gain=0.3  ParamDataTypeStr=single  OutDataTypeStr=single  SaturateOnIntegerOverflow=on
  Demux : Demux  Outputs=2
  PD Z-axis : Scope  NumInputPorts=2
  P_z : Gain  Gain=0.8  ParamDataTypeStr=single  OutDataTypeStr=single  SaturateOnIntegerOverflow=on
  SaturationThrust : Saturate  UpperLimit=4*Controller.totalThrustMaxRelative*Controller.motorsThrustPerMotorMax  LowerLimit=-4*Controller.totalThrustMaxRelative*Controller.motorsThrustPerMotorMax  OutDataTypeStr=single
  Sum : Sum  Inputs=+-|
  Sum15 : Sum  Inputs=|+-  AccumDataTypeStr=single  OutDataTypeStr=single  SaturateOnIntegerOverflow=on
  Sum3 : Sum  Inputs=+-|  AccumDataTypeStr=single  OutDataTypeStr=single  SaturateOnIntegerOverflow=on
  Sum4 : Sum  Inputs=++|  AccumDataTypeStr=single  OutDataTypeStr=single  SaturateOnIntegerOverflow=on
  w0 : Constant  Value=-g*Vehicle.Airframe.mass  OutDataTypeStr=single  SampleTime=Ts
  altitude_cmd : Outport  VectorParamsAs1DForOutWhenUnconnected=off
  wires:
  Sum3/1 -> P_z/1  "errZ"
  Bus Selector6/1 -> Sum3/2  "<Z>"
  w0/1 -> Sum4/1
  D_z/1 -> Sum15/2  "dz"
  P_z/1 -> Sum15/1
  Sum15/1 -> PD Z-axis/2, Sum4/2
  Sum4/1 -> PD Z-axis/1, SaturationThrust/1
  SaturationThrust/1 -> altitude_cmd/1
  PosZ/1 -> Demux/1
  states_estim/1 -> Bus Selector6/1
  Demux/1 -> Sum3/1
  Sum/1 -> D_z/1
  Bus Selector6/2 -> Sum/2  "<dz>"
  Demux/2 -> Sum/1

== system flightController/Flight Controller/Reference point tracking (X,Y) Plane/Subsystem ==
  Varying ref : Inport
  Selector : Inport  Port=2
  Refference Point : Constant  Value=[0 0 -1.4]  OutDataTypeStr=single
  Switch : Switch  Criteria=u2 > Threshold
  PStar : Outport
  wires:
  Refference Point/1 -> Switch/1
  Switch/1 -> PStar/1
  Selector/1 -> Switch/2
  Varying ref/1 -> Switch/3

== system flightController/Flight Controller/Reference point tracking (X,Y) Plane/Subsystem1 ==
  Selector : Inport
  landing flag : Inport  Port=2
  Constant : Constant  Value=false
  Switch : Switch  Criteria=u2 > Threshold
  PStar : Outport
  wires:
  Constant/1 -> Switch/1
  Switch/1 -> PStar/1
  Selector/1 -> Switch/2
  landing flag/1 -> Switch/3

== system flightController/Flight Controller/Reference point tracking X,Y Plane/Subsystem ==
  Varying ref : Inport
  Selector : Inport  Port=2
  Refference Point : Constant  Value=[0 0 -1.4]
  Switch : Switch  Criteria=u2 > Threshold
  PStar : Outport
  wires:
  Refference Point/1 -> Switch/1
  Switch/1 -> PStar/1
  Selector/1 -> Switch/2
  Varying ref/1 -> Switch/3

== system flightController/Flight Controller/Reference point tracking X,Y Plane/Subsystem1 ==
  Selector : Inport
  landing flag : Inport  Port=2
  Constant : Constant  Value=false
  Switch : Switch  Criteria=u2 > Threshold
  PStar : Outport
  wires:
  Constant/1 -> Switch/1
  Switch/1 -> PStar/1
  Selector/1 -> Switch/2
  landing flag/1 -> Switch/3

== matlab function flightController/Flight Controller/New PD + Vel/Altitude reference manipulation With Velocity calculation/Landing spline Dependent on time - works My version ==
  data: z input; PStarZ output; time input; flag input
function PStarZ= fcn(z, time, flag)
    zLanded = -0.1;
    zContraints = [z 0 zLanded 0]';
    t = 0;
    B0 = [1 t, t^2 t^3];
    BPrime0 = [0 1 2*t 3*t^2];
    
    t = 10;
    B1 = [1 t, t^2 t^3];
    BPrime1 = [0 1 2*t 3*t^2];

    BMat = [    B0;
                BPrime0;
                B1;
                BPrime1     ];
            
    Alpha = inv(BMat)*zContraints;
    
    persistent landed;
    if(isempty(landed))
        landed = 0;
    end
    persistent td;
    if(isempty(td))
       td = 0;
    end
    
    if(flag == true)
        td = td + time;
        P = Alpha'*[1 td td^2 td^3]';
        if(P >= zLanded)
            landed = 1;
        end
        if(landed == 1)
            P = single(zLanded);
        end
    else
        P = z;
    end
PStarZ = P;

== matlab function flightController/Flight Controller/New PD + Vel/Altitude reference manipulation With Velocity calculation/Landing spline Dependent on time - works1 ==
  data: z input; zDot input; ZdOut output; time input; flag input
function ZdOut = fcn(z, zDot, time, flag)
    zLanded = single(-0.4);
    zContraints = [z zDot zLanded 0]';
    t = single(0);
    B0 = [1 t, t^2 t^3];
    BPrime0 = [0 1 2*t 3*t^2];
    
    t = single(10);
    B1 = [1 t, t^2 t^3];
    BPrime1 = [0 1 2*t 3*t^2];

    BMat = [    B0;
                BPrime0;
                B1;
                BPrime1     ];
            
    Alpha = inv(BMat)*zContraints;
    
    persistent landed;
    if(isempty(landed))
        landed = 0;
    end
    persistent td;
    if(isempty(td))
       td = single(0);
    end
    zd = 0;
    zdDot = 0;
    if(flag == true)
        if(landed == 0)
            td = td + time;
            zd = Alpha'*[1 td td^2 td^3]';
            zdDot = Alpha'*[0 1 2*td 3*td^2]';
        else 
            zd = single(zLanded);
            zdDot = single(0);
        end
        if(zd >= zLanded-0.01)
            landed = 1;
        end
    else
        zd = z;
        zdDot = single(zDot);
    end
ZdOut = [zd zdDot];

== matlab function flightController/Flight Controller/Reference point tracking (X,Y) Plane/Point tracking old bad way ==
  data: R input; pStar output; xHat input
function pStar = fcn(R, xHat)
persistent i;
persistent td;
if(isempty(i))
    i = 1;
    td = 0;
end
td = td +1;
wayPoints = [0 0 -0.7; 1 0 -0.7; 0 1 -0.7; -1 0 -0.7; 0 -1 -0.7];
if( R^2 >= ((xHat(1)-wayPoints(i,1))^2+(xHat(2)-wayPoints(i,2)^2)) )
    if(td > 1000)
        i = i+1;
        td = 0;
        if(i > length(wayPoints))
            i = length(wayPoints);
        end
    end
end

pStar = wayPoints(i,:)';

== matlab function flightController/Flight Controller/Reference point tracking (X,Y) Plane/Spline positioning ==
  data: pStar output
function pStar = fcn()
xConstraints = [0 0 0.5 1 0.5 1 1.5 0];
yConstraints = [0 0 1   2 1   2 2   0];

persistent td;
if(isempty(td))
    td = 0;
end
td = td + 1;

sigma = 0;
b0 = [1 sigma sigma^2 sigma^3];
b0p = [0 1 2*sigma 3*sigma^2];

sigma = 10;
b1 = [1 sigma sigma^2 sigma^3];
b1pp = [0 0 2 6*sigma];

sigma = 20;
b2 = [1 sigma sigma^2 sigma^3];
b2p = [0 1 2*sigma 3*sigma^2];

BMat = [    b0   zeros(1,4);
            b0p  zeros(1,4);
            b1   zeros(1,4);
            b1pp zeros(1,4);
            zeros(1,4)   b1;
            zeros(1,4) b1pp;
            zeros(1,4)   b2;
            zeros(1,4)  b2p     ];
x = 0;
y = 0;
xAlpha = inv(BMat)*xConstraints';
yAlpha = inv(BMat)*yConstraints';

if(td <=10)
   x = xAlpha(1:4)'*[1 td td^2 td^3]';
   y = yAlpha(1:4)'*[1 td td^2 td^3]';
end
if(td > 10)
   x = xAlpha(5:8)'*[1 td td^2 td^3]';
   y = yAlpha(5:8)'*[1 td td^2 td^3]';
end

pStar = [x y -0.7]';

== matlab function flightController/Flight Controller/Reference point tracking X,Y Plane/Spline positioning ==
  data: pStar output
function pStar = fcn()
xConstraints = [0 0 0.5 1 0.5 1 1.5 0];
yConstraints = [0 0 1   2 1   2 2   0];

persistent td;
if(isempty(td))
    td = 0;
end
td = td + 1;

sigma = 0;
b0 = [1 sigma sigma^2 sigma^3];
b0p = [0 1 2*sigma 3*sigma^2];

sigma = 10;
b1 = [1 sigma sigma^2 sigma^3];
b1pp = [0 0 2 6*sigma];

sigma = 20;
b2 = [1 sigma sigma^2 sigma^3];
b2p = [0 1 2*sigma 3*sigma^2];

BMat = [    b0   zeros(1,4);
            b0p  zeros(1,4);
            b1   zeros(1,4);
            b1pp zeros(1,4);
            zeros(1,4)   b1;
            zeros(1,4) b1pp;
            zeros(1,4)   b2;
            zeros(1,4)  b2p     ];
x = 0;
y = 0;
xAlpha = inv(BMat)*xConstraints';
yAlpha = inv(BMat)*yConstraints';

if(td <=10)
   x = xAlpha(1:4)'*[1 td td^2 td^3]';
   y = yAlpha(1:4)'*[1 td td^2 td^3]';
end
if(td > 10)
   x = xAlpha(5:8)'*[1 td td^2 td^3]';
   y = yAlpha(5:8)'*[1 td td^2 td^3]';
end

pStar = [x y -0.7]';

== matlab function flightController/Flight Controller/full state lqr - not working/Extract 1,2,3,4 ==
  data: u input; y output
function y = fcn(u)

y = u(1:4);

== matlab function flightController/Flight Controller/Reference point tracking X,Y Plane/Line of sight Guidance ==
  data: pTarget input; pStar output; xHat input; flag input
function pStar = fcn(pTarget, xHat, flag)
% This function generates small intermediate points between the actual position
% and the desired reference point, so that the controller will not be
% overwelmed by having to make a too large motor command that the drone
% cannot take without falling out of the skies.

% Initialize variables
%PxTilte = 0;
%PyTilte = 0;
k = 0.1;

% Calculate position error pTilte
PxTilte = xHat(1)-pTarget(1);
PyTilte = xHat(2)-pTarget(2);

% Calculate pTilte norm
pTilteNorm = sqrt(PxTilte^2+PyTilte^2);

% Velocity in the direction I want from pTiltes
vd_x = -k*(PxTilte/(pTilteNorm));
vd_y = -k*(PyTilte/(pTilteNorm));

if(flag == true)
    vd_x = single(0);
    vd_y = single(0);
end

pStar = [xHat(1)+vd_x xHat(2)+vd_y pTarget(3)]';


% The velocity constantly changes when hovering at a waypoint. 
% This will make the drone oscillate around that point.
% To stop this, the velocity calculation should stop when hovering

== matlab function flightController/Flight Controller/Reference point tracking X,Y Plane/Point tracking ==
  data: R input; pTarget output; xHat input; flag output
function [pTarget, flag]= fcn(R, xHat)
%% This function is only responsible for changing reference point when the 
% drone is within some radius R to the reference point. 
persistent i;
if(isempty(i))
    i = 1;
end
persistent temp;
if(isempty(temp))
    temp = false;
end
wayPoints = [0 0 -0.7; 0 1 -0.7; 1 0 -0.7; 1 1 -1];
if( R^2 >= ((xHat(1)-wayPoints(i,1))^2+(xHat(2)-wayPoints(i,2))^2) )
        i = i+1;
        if(i > length(wayPoints))
            i = length(wayPoints);
            temp = true;
        end
        
end
pTarget = wayPoints(i,:)';
flag = temp;

== matlab function flightController/Flight Controller/full state lqr - not working/MATLAB Function ==
  data: u input; Thrust output; gain input
function Thrust = fcn(u, gain)

Thrust = (((-u(1)-u(2)-u(3)-u(4))*1)*gain);

== matlab function flightController/Flight Controller/Altitude reference manipulation/Landing spline Dependent on time - works ==
  data: z input; ZdOut output; time input; flag input
function ZdOut = fcn(z, time, flag)
    zLanded = single(0);
    zContraints = [z 0 zLanded 0]';
    t = single(0);
    B0 = [1 t, t^2 t^3];
    BPrime0 = [0 1 2*t 3*t^2];
    
    t = max(single(3),single(abs(z)*7));
    B1 = [1 t, t^2 t^3];
    BPrime1 = [0 1 2*t 3*t^2];

    BMat = [    B0;
                BPrime0;
                B1;
                BPrime1     ];
            
    Alpha = inv(BMat)*zContraints;
    
    persistent landed;
    if(isempty(landed))
        landed = 0;
    end
    persistent td;
    if(isempty(td))
       td = single(0);
    end
    zd = 0;
    if(flag == true)
        if(landed == 0)
            td = td + time;
            zd = Alpha'*[1 td td^2 td^3]';
        else 
            zd = single(zLanded);
        end
        if(zd >= zLanded-0.03)
            landed = 1;
        end
    else
        zd = z;
    end
ZdOut = zd;

== matlab function flightController/Flight Controller/Reference point tracking X,Y Plane/Point tracking old bad way ==
  data: R input; pStar output; xHat input
function pStar = fcn(R, xHat)
persistent i;
persistent td;
if(isempty(i))
    i = 1;
    td = 0;
end
td = td +1;
wayPoints = [0 0 -0.7; 1 0 -0.7; 0 1 -0.7; -1 0 -0.7; 0 -1 -0.7];
if( R^2 >= ((xHat(1)-wayPoints(i,1))^2+(xHat(2)-wayPoints(i,2)^2)) )
    if(td > 1000)
        i = i+1;
        td = 0;
        if(i > length(wayPoints))
            i = length(wayPoints);
        end
    end
end

pStar = wayPoints(i,:)';

== matlab function flightController/Flight Controller/Altitude reference manipulation/Landing spline Dependent on time - works My version ==
  data: z input; PStarZ output; time input; flag input
function PStarZ= fcn(z, time, flag)
    zLanded = -0.1;
    zContraints = [z 0 zLanded 0]';
    t = 0;
    B0 = [1 t, t^2 t^3];
    BPrime0 = [0 1 2*t 3*t^2];
    
    t = 10;
    B1 = [1 t, t^2 t^3];
    BPrime1 = [0 1 2*t 3*t^2];

    BMat = [    B0;
                BPrime0;
                B1;
                BPrime1     ];
            
    Alpha = inv(BMat)*zContraints;
    
    persistent landed;
    if(isempty(landed))
        landed = 0;
    end
    persistent td;
    if(isempty(td))
       td = 0;
    end
    
    if(flag == true)
        td = td + time;
        P = Alpha'*[1 td td^2 td^3]';
        if(P >= zLanded)
            landed = 1;
        end
        if(landed == 1)
            P = single(zLanded);
        end
    else
        P = z;
    end
PStarZ = P;

== matlab function flightController/Flight Controller/Reference point tracking (X,Y) Plane/Line of sight Guidance ==
  data: pTarget input; pStar output; xHat input; landFlag input; markerFlag input; marker input
function pStar = fcn(pTarget, xHat, landFlag, markerFlag, marker)
% This function generates small intermediate points between the actual position
% and the desired reference point, so that the controller will not be
% overwelmed by having to make a too large motor command that the drone
% cannot take without falling out of the skies.

% Initialize variables
%PxTilte = 0;
%PyTilte = 0;
k = 0.1;

% Calculate position error pTilte
PxTilte = xHat(1)-pTarget(1);
PyTilte = xHat(2)-pTarget(2);

% Calculate pTilte norm
pTilteNorm = sqrt(PxTilte^2+PyTilte^2);

% Velocity in the direction I want from pTilte
vd_x = -k*(PxTilte/(pTilteNorm));
vd_y = -k*(PyTilte/(pTilteNorm));

if(landFlag == true)
    if(abs(PxTilte)<0.1)
        vd_x = single(0);
    end
    if(abs(PyTilte)<0.1)
        vd_y = single(0);
    end
end
if(markerFlag == true)
    vd_x = (vd_x*abs(marker(1)*2));
    vd_y = (vd_y*abs(marker(2)*2));
    if abs(PxTilte) < 0.00001
        vd_x = single(0);
    end
    if abs(PyTilte) < 0.00001
        vd_y = single(0);
    end
end
pStar = [xHat(1)+vd_x xHat(2)+vd_y pTarget(3)]';

% The velocity constantly changes when hovering at a waypoint. 
% This will make the drone oscillate around that point.
% To stop this, the velocity calculation should stop when hovering

== matlab function flightController/Flight Controller/Reference point tracking (X,Y) Plane/Point tracking ==
  data: R input; pTarget output; xHat input; LandingFlag output; marker input; markerFlag output
function [pTarget, LandingFlag, markerFlag]= fcn(R, xHat, marker)
%% This function is only responsible for changing reference point when the 
% drone is within some radius R to the reference point. 
%% Variables
persistent i;
if(isempty(i))
    i = 1;
end
persistent temp;
if(isempty(temp))
    temp = false;
end

persistent markerTemp;
if(isempty(markerTemp))
    markerTemp = false;
end
% The drone does not like going above 2m...
wayPoints = [0 0 -1.5; 1 0 -1.5; 1 1 -1.5; 0 2 -1.5; -1 1 -1.5; -2 0 -1.5; -1 -1 -1.5; 0 -2 -1.5; 1 -1 -1.5];
%wayPoints = [0 0 -1.2; 1 0 -.5; 1 -1 -2];
if( marker(1) == 0 && marker(2) == 0 && markerTemp == false)
    %% Waypoint shifting
    if( R^2 >= ((xHat(1)-wayPoints(i,1))^2 +(xHat(2)-wayPoints(i,2))^2) && R >=(abs(xHat(3))-abs(wayPoints(i,3))))
            i = i+1;
            if(i > length(wayPoints))
                i = length(wayPoints);
                temp = true;
            end
    end
else
        markerTemp = true;
        wayPoints(i,1) = (xHat(1)+marker(1)*-1);
        wayPoints(i,2) = (xHat(2)+marker(2));
end

%% Create output
pTarget = wayPoints(i,:)';
LandingFlag = temp;
markerFlag = markerTemp;
